simulink model "S12_V8_Muscle_v10"  (R2026a)
settings: Solver=FixedStepDiscrete  StopTime=89.98  FixedStep=0.02
model workspace (MAT data in the model file):
  v10_acceleration_gain = 0.32
  v10_area_m2 = 0.03
  v10_attack = 0.25
  v10_backfire = timeseries
  v10_backfire.Name = 'unnamed'
  v10_backfire.DataInfo = tsdata.datametadata
  v10_backfire.DataInfo.Interpolation = tsdata.interpolation
  v10_backfire.DataInfo.Interpolation.Fhandle : function handle (value not decoded)
  v10_backfire.DataInfo.Interpolation.Name = 'linear'
  v10_backfire.TimeInfo = tsdata.timemetadata
  v10_backfire.TimeInfo.Length = 4500
  v10_backfire.TimeInfo.DuplicateTimes = 0
  v10_backfire.TimeInfo.Time_ = [0 0.02 0.04 0.06 0.08 0.1 0.12 0.14 0.16 0.18 0.2 0.22 ... (4500 elements, 4500x1)]
  v10_backfire.TimeInfo.Initialized = 1
  v10_backfire.QualityInfo = tsdata.qualmetadata
  v10_backfire.Data_ = [0 0 0 0 0 0 0 0 0 0 0 0 ... (4500 elements, 4500x1)]
  v10_bank_map = [1 2 1 1 2 2 2 1]
  v10_cylinder_count = 8
  v10_damping = 0.11
  v10_dashboard_acceleration = 0
  v10_dashboard_backfire_scale = 1
  v10_dashboard_load = 0.1
  v10_dashboard_order_balance = 1
  v10_dashboard_overrun = 0
  v10_dashboard_rpm = 700
  v10_dashboard_speed_kph = 0
  v10_dashboard_throttle = 0.1
  v10_dashboard_transient_scale = 1
  v10_decay = 0.82
  v10_firing_order = [1 8 4 3 6 5 7 2]
  v10_firing_phase_deg = [0 90 180 270 360 450 540 630]
  v10_gain_db = -15
  v10_harmonic_tilt = 0.55
  v10_intake_tone = 0.25
  v10_interactive_mode = 0
  v10_lift_gain = 0.26
  v10_order_gains = [1 0.82 0.64 0.44 0.3 0.2]
  v10_pipe_length_m = 1.9
  v10_profile_id = "hellcat_style_supercharged_v8"
  v10_pulse_sharpness = 0.82
  v10_reflection = 0.44
  v10_reset = timeseries
  v10_reset.Name = 'unnamed'
  v10_reset.DataInfo = tsdata.datametadata
  v10_reset.DataInfo.Interpolation = tsdata.interpolation
  v10_reset.DataInfo.Interpolation.Fhandle : function handle (value not decoded)
  v10_reset.DataInfo.Interpolation.Name = 'linear'
  v10_reset.TimeInfo = tsdata.timemetadata
  v10_reset.TimeInfo.Length = 4500
  v10_reset.TimeInfo.DuplicateTimes = 0
  v10_reset.TimeInfo.Time_ = [0 0.02 0.04 0.06 0.08 0.1 0.12 0.14 0.16 0.18 0.2 0.22 ... (4500 elements, 4500x1)]
  v10_reset.TimeInfo.Initialized = 1
  v10_reset.QualityInfo = tsdata.qualmetadata
  v10_reset.Data_ = [1 0 0 0 0 0 0 0 0 0 0 0 ... (4500 elements, 4500x1)]
  v10_supercharger_tone = 0.32
  v10_vehicle_state = timeseries
  v10_vehicle_state.Name = 'unnamed'
  v10_vehicle_state.DataInfo = tsdata.datametadata
  v10_vehicle_state.DataInfo.Interpolation = tsdata.interpolation
  v10_vehicle_state.DataInfo.Interpolation.Fhandle : function handle (value not decoded)
  v10_vehicle_state.DataInfo.Interpolation.Name = 'linear'
  v10_vehicle_state.TimeInfo = tsdata.timemetadata
  v10_vehicle_state.TimeInfo.Length = 4500
  v10_vehicle_state.TimeInfo.DuplicateTimes = 0
  v10_vehicle_state.TimeInfo.Time_ = [0 0.02 0.04 0.06 0.08 0.1 0.12 0.14 0.16 0.18 0.2 0.22 ... (4500 elements, 4500x1)]
  v10_vehicle_state.TimeInfo.Initialized = 1
  v10_vehicle_state.QualityInfo = tsdata.qualmetadata
  v10_vehicle_state.Data_ = [700 700 700 700 700 700 700 700 700 700 700 700 ... (27000 elements, 4500x6)]
settings Model: Creator=Jovi  LastModifiedBy=Jovi

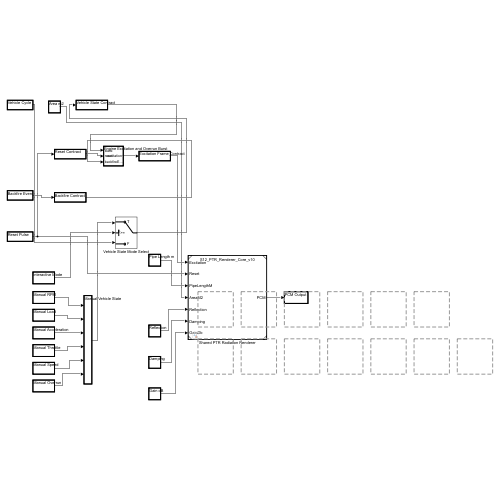
[thumbnail: Simulink's stored preview of the top-level diagram]
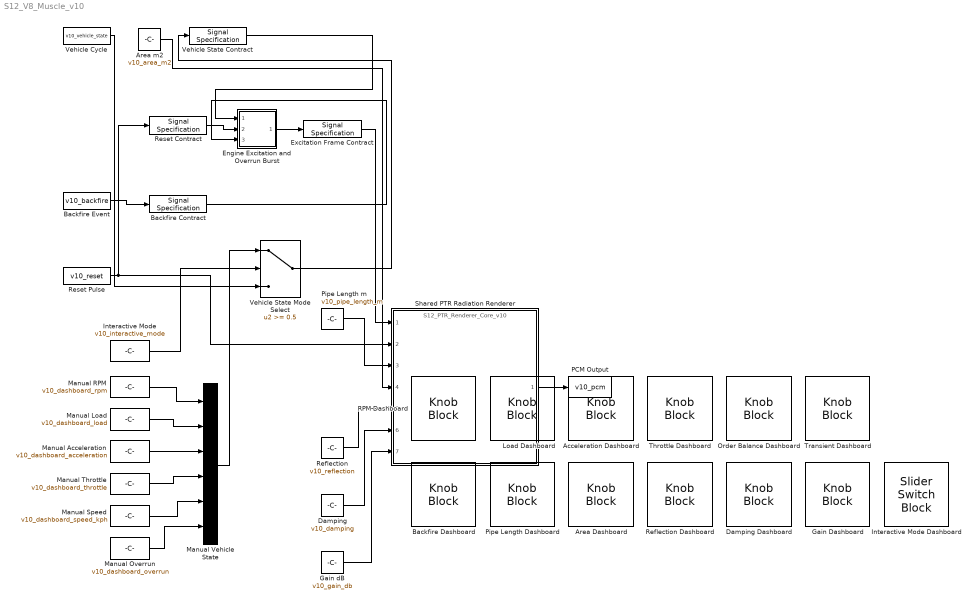
== system S12_V8_Muscle_v10 ==
  Acceleration Dashboard : KnobBlock  ShowInitialText=off  ScaleMin=-5  ScaleMax=8
  Area Dashboard : KnobBlock  ShowInitialText=off  ScaleMin=0.0050000000000000001  ScaleMax=0.10000000000000001
  Area m2 : Constant  Value=v10_area_m2
  Backfire Contract : SignalSpecification  OutDataTypeStr=double  Dimensions=1  SampleTime=0.02
  Backfire Dashboard : KnobBlock  ShowInitialText=off  ScaleMax=2
  Backfire Event : FromWorkspace  VariableName=v10_backfire  OutDataTypeStr=double  SampleTime=0.02
  Damping : Constant  Value=v10_damping
  Damping Dashboard : KnobBlock  ShowInitialText=off  ScaleMin=0.001  ScaleMax=0.29999999999999999
  Engine Excitation and Overrun Burst : MATLAB Function  TreatAsAtomicUnit=on
  Excitation Frame Contract : SignalSpecification  OutDataTypeStr=double  Dimensions=[960 1]  SampleTime=0.02
  Gain Dashboard : KnobBlock  ShowInitialText=off  ScaleMin=-30  ScaleMax=6
  Gain dB : Constant  Value=v10_gain_db
  Interactive Mode : Constant  Value=v10_interactive_mode  OutDataTypeStr=boolean  SampleTime=0.02
  Interactive Mode Dashboard : SliderSwitchBlock  ShowInitialText=off
  Load Dashboard : KnobBlock  ShowInitialText=off  ScaleMax=1
  Manual Acceleration : Constant  Value=v10_dashboard_acceleration  SampleTime=0.02
  Manual Load : Constant  Value=v10_dashboard_load  SampleTime=0.02
  Manual Overrun : Constant  Value=v10_dashboard_overrun  SampleTime=0.02
  Manual RPM : Constant  Value=v10_dashboard_rpm  SampleTime=0.02
  Manual Speed : Constant  Value=v10_dashboard_speed_kph  SampleTime=0.02
  Manual Throttle : Constant  Value=v10_dashboard_throttle  SampleTime=0.02
  Manual Vehicle State : Mux  Inputs=6
  Order Balance Dashboard : KnobBlock  ShowInitialText=off  ScaleMax=2
  PCM Output : ToWorkspace  VariableName=v10_pcm  SaveFormat=Structure With Time  SampleTime=0.02
  Pipe Length Dashboard : KnobBlock  ShowInitialText=off  ScaleMin=0.40000000000000002  ScaleMax=4
  Pipe Length m : Constant  Value=v10_pipe_length_m
  RPM Dashboard : KnobBlock  ShowInitialText=off  ScaleMin=500  ScaleMax=10000
  Reflection : Constant  Value=v10_reflection
  Reflection Dashboard : KnobBlock  ShowInitialText=off  ScaleMax=0.98999999999999999
  Reset Contract : SignalSpecification  OutDataTypeStr=boolean  Dimensions=1  SampleTime=0.02
  Reset Pulse : FromWorkspace  VariableName=v10_reset  OutDataTypeStr=boolean  SampleTime=0.02
  Shared PTR Radiation Renderer : ModelReference  ModelNameDialog=S12_PTR_Renderer_Core_v10  SimulationMode=Normal  ModelReferenceVersion=1.3
  Throttle Dashboard : KnobBlock  ShowInitialText=off  ScaleMax=1
  Transient Dashboard : KnobBlock  ShowInitialText=off  ScaleMax=2
  Vehicle Cycle : FromWorkspace  VariableName=v10_vehicle_state  OutDataTypeStr=double  SampleTime=0.02
  Vehicle State Contract : SignalSpecification  OutDataTypeStr=double  Dimensions=6  SampleTime=0.02
  Vehicle State Mode Select : Switch  Threshold=0.5
  wires:
  Vehicle State Contract/1 -> Engine Excitation and Overrun Burst/1(state)
  Reset Pulse/1 -> Shared PTR Radiation Renderer/2, Reset Contract/1
  Reset Contract/1 -> Engine Excitation and Overrun Burst/2(reset)
  Backfire Event/1 -> Backfire Contract/1
  Backfire Contract/1 -> Engine Excitation and Overrun Burst/3(backfireEnergy)
  Engine Excitation and Overrun Burst/1(excitation) -> Excitation Frame Contract/1
  Excitation Frame Contract/1 -> Shared PTR Radiation Renderer/1
  Pipe Length m/1 -> Shared PTR Radiation Renderer/3
  Area m2/1 -> Shared PTR Radiation Renderer/4
  Reflection/1 -> Shared PTR Radiation Renderer/5
  Damping/1 -> Shared PTR Radiation Renderer/6
  Gain dB/1 -> Shared PTR Radiation Renderer/7
  Shared PTR Radiation Renderer/1 -> PCM Output/1
  Manual RPM/1 -> Manual Vehicle State/1
  Manual Load/1 -> Manual Vehicle State/2
  Manual Acceleration/1 -> Manual Vehicle State/3
  Manual Throttle/1 -> Manual Vehicle State/4
  Manual Speed/1 -> Manual Vehicle State/5
  Manual Overrun/1 -> Manual Vehicle State/6
  Manual Vehicle State/1 -> Vehicle State Mode Select/1
  Interactive Mode/1 -> Vehicle State Mode Select/2
  Vehicle Cycle/1 -> Vehicle State Mode Select/3
  Vehicle State Mode Select/1 -> Vehicle State Contract/1

== matlab function S12_V8_Muscle_v10/Engine Excitation and Overrun Burst ==
  data: state input; excitation output double size=[960 1]; reset input; backfireEnergy input; v10_cylinder_count parameter double size=1; v10_firing_order parameter double size=[1 8]; v10_firing_phase_deg parameter double size=[1 8]; v10_bank_map parameter double size=[1 8]; v10_order_gains parameter double size=[1 6]; v10_pulse_sharpness parameter double size=1; v10_harmonic_tilt parameter double size=1; v10_intake_tone parameter double size=1; v10_supercharger_tone parameter double size=1; v10_attack parameter double size=1; v10_decay parameter double size=1; v10_acceleration_gain parameter double size=1; v10_lift_gain parameter double size=1; v10_dashboard_order_balance parameter double size=1; v10_dashboard_transient_scale parameter double size=1; v10_dashboard_backfire_scale parameter double size=1
function excitation = fcn(state, reset, backfireEnergy, v10_cylinder_count, v10_firing_order, v10_firing_phase_deg, v10_bank_map, v10_order_gains, v10_pulse_sharpness, v10_harmonic_tilt, v10_intake_tone, v10_supercharger_tone, v10_attack, v10_decay, v10_acceleration_gain, v10_lift_gain, v10_dashboard_order_balance, v10_dashboard_transient_scale, v10_dashboard_backfire_scale)
%#codegen
excitation = s12_engine_sound_model_excitation_step(state, reset, v10_cylinder_count, v10_firing_order, v10_firing_phase_deg, v10_bank_map, v10_order_gains * v10_dashboard_order_balance, v10_pulse_sharpness, v10_harmonic_tilt, v10_intake_tone, v10_supercharger_tone, v10_attack * v10_dashboard_transient_scale, v10_decay, v10_acceleration_gain * v10_dashboard_transient_scale, v10_lift_gain * v10_dashboard_transient_scale, backfireEnergy * v10_dashboard_backfire_scale);
end
